simulink model "ChevNAOcorrection"  (R2015b)
settings: Solver=ode45  StartTime=0.0  StopTime=1  MaxStep=0.01  RelTol=1e-3
values from neighbouring files (symbols this model uses):
  Cext = 0    [ParamChev.m]
  f = 1.6E-5    (= 1.6e-05)    [ParamChev.m]
  Jeq = Jmot + Jch*k^2    (= 8.25325812238e-06)    [ParamChev.m]
  k = 13*25*12*10/(80*47*58*36)    (= 0.00496759598924)    [ParamChev.m]
  Ke = 0.0194    [ParamChev.m]
  Ki = 0.0194    [ParamChev.m]
  R = 5.4    [ParamChev.m]
  Vbat = 24    [ParamChev.m]
undefined symbols (not defined in the file or in its folder): Kd, Kp
settings Model: Creator=antomart  LastModifiedBy=David
settings DataIOCC: LimitDataPoints=off  SaveFormat=StructureWithTime
settings HardwareCC: ProdWordSize=32  ProdHWDeviceType=Specified
settings ModelReferenceCC: PropagateSignalLabelsOutOfModel=on
settings GRTTargetCC: GeneratePreprocessorConditionals=Disable all

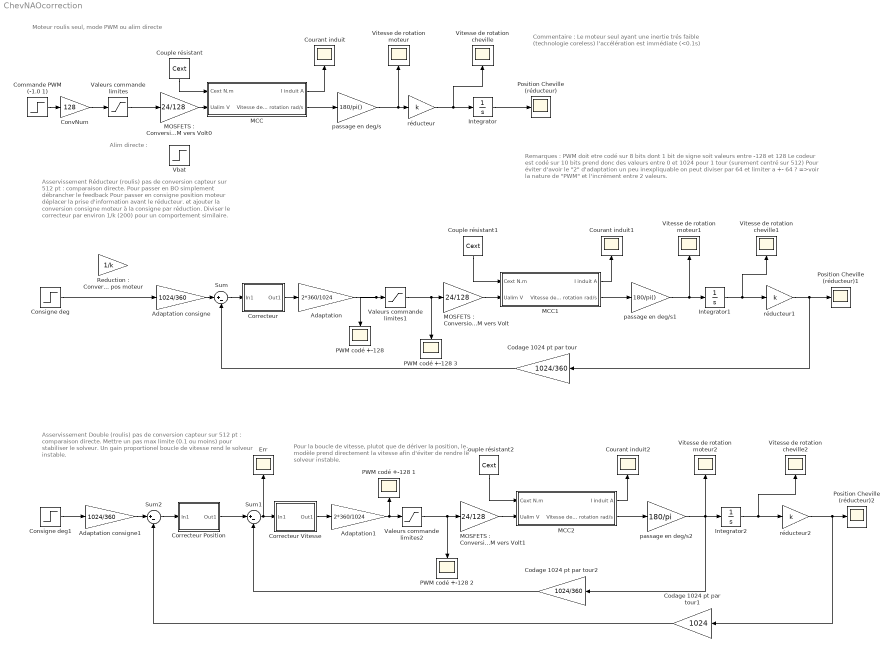
== system ChevNAOcorrection ==
  note: Pour la boucle de vitesse, plutot que de dériver la position,
      |  le modèle prend directement la vitesse
      | afin d'éviter de rendre le solveur instable.
  note: Remarques : PWM doit etre codé sur 8 bits dont 1 bit de signe soit valeurs entre -128 et 128
      | Le codeur est codé sur 10 bits  prend donc des valeurs entre 0 et 1024 pour 1 tour (surement centré sur 512)
      | Pour éviter d'avoir le "2" d'adaptation un peu inexpliquable on peut diviser par 64 et limiter a +- 64 ?
      | =>voir la nature de "PWM" et l'incrément entre 2 valeurs.
  note: Alim directe :
  note: Asservissement Réducteur (roulis)
      | pas de conversion capteur sur 512 pt : comparaison directe.
      | Pour passer en BO simplement débrancher le feedback
      | Pour passer en consigne position moteur
      | déplacer la prise d'information avant le réducteur. et ajouter
      | la conversion consigne moteur à la consigne par réduction.
      | Diviser le correcteur par environ 1/k (200)
      | pour un comportement similaire.
  note: Moteur roulis seul, mode PWM ou alim directe
  note: Commentaire :
      | Le moteur seul ayant une inertie trés faible
      | (technologie coreless) l'accélération est immédiate (<0.1s)
  note: Asservissement Double (roulis)
      | pas de conversion capteur sur 512 pt : comparaison directe.
      | Mettre un pas max limite (0.1 ou moins) pour stabiliser le solveur.
      | Un gain proportionel boucle de vitesse rend le solveur instable.
  Adaptation : Gain  Gain=2*360/1024
  Adaptation consigne : Gain  Gain=1024/360
  Adaptation consigne1 : Gain  Gain=1024/360
  Adaptation1 : Gain  Gain=2*360/1024
  Codage 1024 pt par tour : Gain  Gain=1024/360
  Codage 1024 pt par tour1 : Gain  Gain=1024
  Codage 1024 pt par tour2 : Gain  Gain=1024/360
  Commande PWM (-1.0 1) : Step  Time=0  After=0.5  SampleTime=0
  Consigne deg : Step  Time=0  After=30  SampleTime=0
  Consigne deg1 : Step  Time=0  After=30  SampleTime=0
  ConvNum : Gain  Gain=128
  Correcteur : Subsystem
  Correcteur Position : Subsystem
  Correcteur Vitesse : Subsystem
  Couple résistant : Constant  Value=Cext
  Couple résistant1 : Constant  Value=Cext
  Couple résistant2 : Constant  Value=Cext
  Courant induit : Scope
  Courant induit1 : Scope
  Courant induit2 : Scope
  Err : Scope
  Integrator : Integrator
  Integrator1 : Integrator
  Integrator2 : Integrator
  MCC : Subsystem
  MCC1 : Subsystem
  MCC2 : Subsystem
  "MOSFETS : Conversion PWM vers Volt" : Gain  Gain=24/128
  "MOSFETS : Conversion PWM vers Volt0" : Gain  Gain=24/128
  "MOSFETS : Conversion PWM vers Volt1" : Gain  Gain=24/128
  PWM codé +-128 1 : Scope
  PWM codé +-128 2 : Scope
  PWM codé +-128 3 : Scope
  PWM codé +-128 : Scope
  Position Cheville (réducteur) : Scope
  Position Cheville (réducteur)1 : Scope
  Position Cheville (réducteur)2 : Scope
  "Reduction : Conversion pos moteur" : Gain  Gain=1/k
  Sum : Sum  Inputs=|+-
  Sum1 : Sum  Inputs=|+-
  Sum2 : Sum  Inputs=|+-
  Valeurs commande limites : Saturate  UpperLimit=128  LowerLimit=-128
  Valeurs commande limites1 : Saturate  UpperLimit=128  LowerLimit=-128
  Valeurs commande limites2 : Saturate  UpperLimit=128  LowerLimit=-128
  Vbat : Step  Time=0  After=Vbat  SampleTime=0
  Vitesse de rotation cheville : Scope
  Vitesse de rotation cheville1 : Scope
  Vitesse de rotation cheville2 : Scope
  Vitesse de rotation moteur : Scope
  Vitesse de rotation moteur1 : Scope
  Vitesse de rotation moteur2 : Scope
  passage en deg/s : Gain  Gain=180/pi()
  passage en deg/s1 : Gain  Gain=180/pi()
  passage en deg/s2 : Gain  Gain=180/pi
  réducteur : Gain  Gain=k
  réducteur1 : Gain  Gain=k
  réducteur2 : Gain  Gain=k
  wires:
  Couple résistant/1 -> MCC/1(Cext N.m)
  MCC/1(I induit A) -> Courant induit/1
  MCC/2(Vitesse de rotation rad/s) -> passage en deg/s/1
  passage en deg/s/1 -> réducteur/1, Vitesse de rotation moteur/1
  réducteur/1 -> Integrator/1, Vitesse de rotation cheville/1
  Couple résistant1/1 -> MCC1/1(Cext N.m)
  MCC1/1(I induit A) -> Courant induit1/1
  MCC1/2(Vitesse de rotation rad/s) -> passage en deg/s1/1
  passage en deg/s1/1 -> Integrator1/1, Vitesse de rotation moteur1/1
  Integrator/1 -> Position Cheville (réducteur)/1
  Integrator1/1 -> réducteur1/1, Vitesse de rotation cheville1/1
  réducteur1/1 -> Codage 1024 pt par tour/1, Position Cheville (réducteur)1/1
  "MOSFETS : Conversion PWM vers Volt0"/1 -> MCC/2(Ualim V)
  Valeurs commande limites/1 -> "MOSFETS : Conversion PWM vers Volt0"/1
  Valeurs commande limites1/1 -> PWM codé +-128 3/1, "MOSFETS : Conversion PWM vers Volt"/1
  "MOSFETS : Conversion PWM vers Volt"/1 -> MCC1/2(Ualim V)
  Sum/1 -> Correcteur/1(In1)
  Correcteur/1(Out1) -> Adaptation/1
  Adaptation/1 -> PWM codé +-128/1, Valeurs commande limites1/1
  Consigne deg/1 -> Adaptation consigne/1
  Couple résistant2/1 -> MCC2/1(Cext N.m)
  MCC2/1(I induit A) -> Courant induit2/1
  MCC2/2(Vitesse de rotation rad/s) -> passage en deg/s2/1
  passage en deg/s2/1 -> Codage 1024 pt par tour2/1, Integrator2/1, Vitesse de rotation moteur2/1
  Integrator2/1 -> réducteur2/1, Vitesse de rotation cheville2/1
  réducteur2/1 -> Codage 1024 pt par tour1/1, Position Cheville (réducteur)2/1
  Valeurs commande limites2/1 -> PWM codé +-128 2/1, "MOSFETS : Conversion PWM vers Volt1"/1
  "MOSFETS : Conversion PWM vers Volt1"/1 -> MCC2/2(Ualim V)
  Sum1/1 -> Correcteur Vitesse/1(In1), Err/1
  Correcteur Vitesse/1(Out1) -> Adaptation1/1
  Adaptation1/1 -> PWM codé +-128 1/1, Valeurs commande limites2/1
  Sum2/1 -> Correcteur Position/1(In1)
  Correcteur Position/1(Out1) -> Sum1/1
  Consigne deg1/1 -> Adaptation consigne1/1
  Commande PWM (-1.0 1)/1 -> ConvNum/1
  ConvNum/1 -> Valeurs commande limites/1
  Codage 1024 pt par tour/1 -> Sum/2
  Adaptation consigne/1 -> Sum/1
  Codage 1024 pt par tour1/1 -> Sum2/2
  Adaptation consigne1/1 -> Sum2/1
  Codage 1024 pt par tour2/1 -> Sum1/2

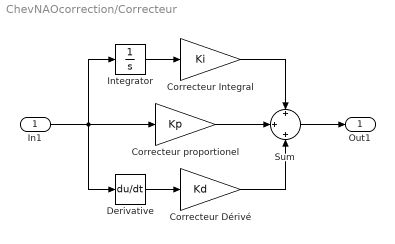
== system ChevNAOcorrection/Correcteur ==
  In1 : Inport
  Correcteur Dérivé : Gain  Gain=Kd
  Correcteur Integral : Gain  Gain=Ki
  Correcteur proportionel : Gain  Gain=Kp
  Derivative : Derivative
  Integrator : Integrator
  Sum : Sum  Inputs=+|+|+
  Out1 : Outport
  wires:
  In1/1 -> Derivative/1, Integrator/1, Correcteur proportionel/1
  Integrator/1 -> Correcteur Integral/1
  Correcteur Integral/1 -> Sum/1
  Correcteur proportionel/1 -> Sum/2
  Derivative/1 -> Correcteur Dérivé/1
  Correcteur Dérivé/1 -> Sum/3
  Sum/1 -> Out1/1

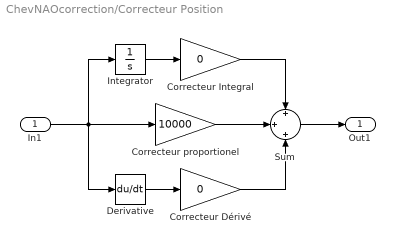
== system ChevNAOcorrection/Correcteur Position ==
  In1 : Inport
  Correcteur Dérivé : Gain  Gain=0
  Correcteur Integral : Gain  Gain=0
  Correcteur proportionel : Gain  Gain=10000
  Derivative : Derivative
  Integrator : Integrator
  Sum : Sum  Inputs=+|+|+
  Out1 : Outport
  wires:
  In1/1 -> Derivative/1, Integrator/1, Correcteur proportionel/1
  Integrator/1 -> Correcteur Integral/1
  Correcteur Integral/1 -> Sum/1
  Correcteur proportionel/1 -> Sum/2
  Derivative/1 -> Correcteur Dérivé/1
  Correcteur Dérivé/1 -> Sum/3
  Sum/1 -> Out1/1

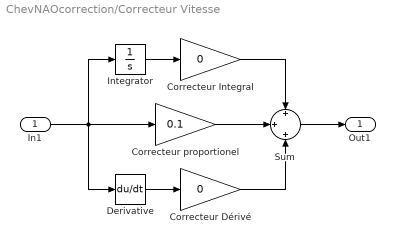
== system ChevNAOcorrection/Correcteur Vitesse ==
  In1 : Inport
  Correcteur Dérivé : Gain  Gain=0
  Correcteur Integral : Gain  Gain=0
  Correcteur proportionel : Gain  Gain=0.1
  Derivative : Derivative
  Integrator : Integrator
  Sum : Sum  Inputs=+|+|+
  Out1 : Outport
  wires:
  In1/1 -> Derivative/1, Integrator/1, Correcteur proportionel/1
  Integrator/1 -> Correcteur Integral/1
  Correcteur Integral/1 -> Sum/1
  Correcteur proportionel/1 -> Sum/2
  Sum/1 -> Out1/1
  Derivative/1 -> Correcteur Dérivé/1
  Correcteur Dérivé/1 -> Sum/3

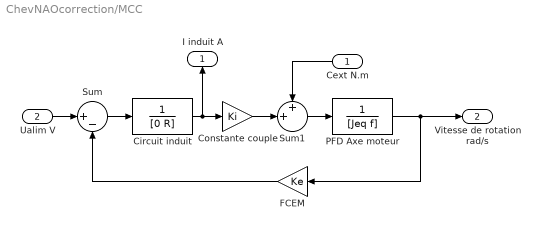
== system ChevNAOcorrection/MCC ==
  Cext N.m : Inport
  Ualim V : Inport  Port=2
  Circuit induit : TransferFcn  Denominator=[0 R]
  Constante couple : Gain  Gain=Ki
  FCEM : Gain  Gain=Ke
  PFD Axe moteur : TransferFcn  Denominator=[Jeq f]
  Sum : Sum  Inputs=|+-
  Sum1 : Sum  Inputs=++|
  I induit A : Outport
  Vitesse de rotation rad/s : Outport  Port=2
  wires:
  PFD Axe moteur/1 -> Vitesse de rotation rad/s/1, FCEM/1
  Sum1/1 -> PFD Axe moteur/1
  Constante couple/1 -> Sum1/2
  Circuit induit/1 -> Constante couple/1, I induit A/1
  Sum/1 -> Circuit induit/1
  FCEM/1 -> Sum/2
  Cext N.m/1 -> Sum1/1
  Ualim V/1 -> Sum/1

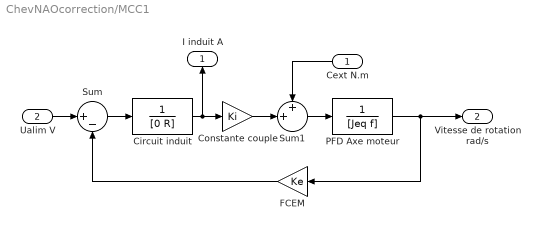
== system ChevNAOcorrection/MCC1 ==
  Cext N.m : Inport
  Ualim V : Inport  Port=2
  Circuit induit : TransferFcn  Denominator=[0 R]
  Constante couple : Gain  Gain=Ki
  FCEM : Gain  Gain=Ke
  PFD Axe moteur : TransferFcn  Denominator=[Jeq f]
  Sum : Sum  Inputs=|+-
  Sum1 : Sum  Inputs=++|
  I induit A : Outport
  Vitesse de rotation rad/s : Outport  Port=2
  wires:
  PFD Axe moteur/1 -> Vitesse de rotation rad/s/1, FCEM/1
  Sum1/1 -> PFD Axe moteur/1
  Constante couple/1 -> Sum1/2
  Circuit induit/1 -> Constante couple/1, I induit A/1
  Sum/1 -> Circuit induit/1
  FCEM/1 -> Sum/2
  Cext N.m/1 -> Sum1/1
  Ualim V/1 -> Sum/1

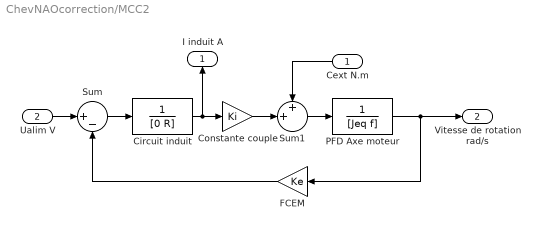
== system ChevNAOcorrection/MCC2 ==
  Cext N.m : Inport
  Ualim V : Inport  Port=2
  Circuit induit : TransferFcn  Denominator=[0 R]
  Constante couple : Gain  Gain=Ki
  FCEM : Gain  Gain=Ke
  PFD Axe moteur : TransferFcn  Denominator=[Jeq f]
  Sum : Sum  Inputs=|+-
  Sum1 : Sum  Inputs=++|
  I induit A : Outport
  Vitesse de rotation rad/s : Outport  Port=2
  wires:
  PFD Axe moteur/1 -> Vitesse de rotation rad/s/1, FCEM/1
  Sum1/1 -> PFD Axe moteur/1
  Constante couple/1 -> Sum1/2
  Circuit induit/1 -> Constante couple/1, I induit A/1
  Sum/1 -> Circuit induit/1
  FCEM/1 -> Sum/2
  Cext N.m/1 -> Sum1/1
  Ualim V/1 -> Sum/1
